simulink model "modelo1"  (R2018a)
settings: Solver=FixedStepAuto  StartTime=0.0  StopTime=0.05  FixedStep=0.0001  RelTol=1e-3
values from neighbouring files (symbols this model uses):
  A = [0 0 1 0;0 0 0 1;k 0 0 x;0 k -x 0]    [autovalores.m]    (also in graficoim.m = 0.0004; sim1.m = [zeros(2) eye(2);Ke*eye(2) -Ge]; sim2.m = [zeros(2) eye(2);Ke*eye(2) -Ge])
  B = kb*[zeros(2);eye(2)]    [autovalores.m]    (also in sim1.m = (1/J)*d*b*ki*[zeros(2);eye(2)]; sim2.m = (1/J)*d*b*ki*[zeros(2);eye(2)])
  C = [eye(2) zeros(2)]    [autovalores.m]    (also in sim1.m; sim2.m)
  F = Fdn    [sim1.m]    (also in sim2.m)
  x0 = [0.0002;-0.0002;0;0]    [sim1.m]    (also in sim2.m)
undefined symbols (not defined in the file or in its folder): L
settings Model: Creator=vinic  LastModifiedBy=vinic

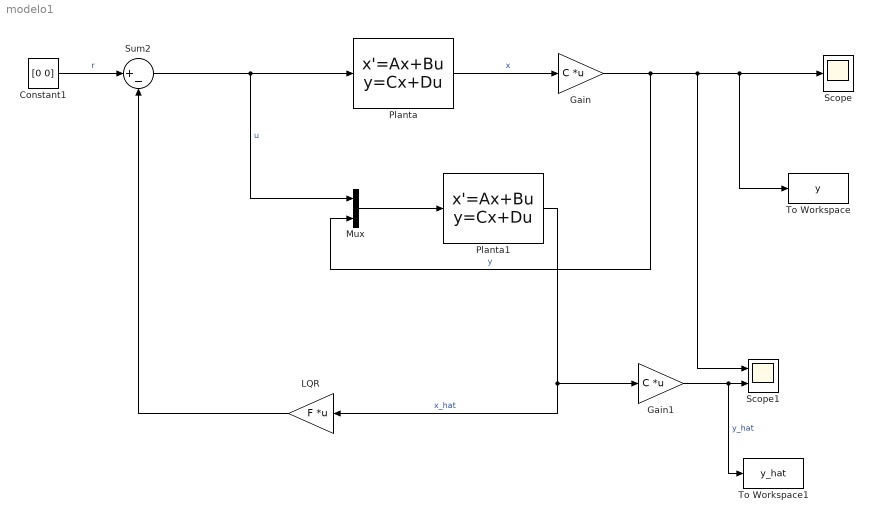
== system modelo1 ==
  Constant1 : Constant  Value=[0 0]
  Gain : Gain  Gain=C  Multiplication=Matrix(K*u)
  Gain1 : Gain  Gain=C  Multiplication=Matrix(K*u)
  LQR : Gain  Gain=F  Multiplication=Matrix(K*u)
  Mux : Mux  Inputs=2
  Planta : StateSpace  A=A  B=B  C=eye(4)  D=zeros(4,2)  InitialCondition=x0
  Planta1 : StateSpace  A=A-L*C  B=[B L]  C=eye(4)  D=zeros(4,4)  InitialCondition=[0;0;0;0]
  Scope : Scope
  Scope1 : Scope  NumInputPorts=2
  Sum2 : Sum  Inputs=|+-
  To Workspace : ToWorkspace  VariableName=y  SampleTime=-1
      settings: Save2DSignal=2-D array (concatenate along first dimension)
  To Workspace1 : ToWorkspace  VariableName=y_hat  SampleTime=-1
      settings: Save2DSignal=2-D array (concatenate along first dimension)
  wires:
  Planta/1 -> Gain/1  "x"
  LQR/1 -> Sum2/2
  Gain/1 -> Scope1/1, To Workspace/1, Scope/1, Mux/2  "y"
  Constant1/1 -> Sum2/1  "r"
  Sum2/1 -> Planta/1, Mux/1  "u"
  Planta1/1 -> Gain1/1, LQR/1  "x_hat"
  Mux/1 -> Planta1/1
  Gain1/1 -> To Workspace1/1, Scope1/2  "y_hat"
